simulink model "HW5_Q1_2sl"  (R2021b)
settings: Solver=VariableStepAuto  StartTime=0.0  StopTime=10.0  RelTol=1e-3
values from neighbouring files (symbols this model uses):
  Bm = 1*10^-5    (= 1e-05)    [HW5_Group3_1_1.m]    (also in HW5_Group3_1_2.m = 1e-08)
  Jm = 3*10^-5    (= 3e-05)    [HW5_Group3_1_1.m]    (also in HW5_Group3_1_2.m = 2.5e-05)
  Km = 3*10^-2    (= 0.03)    [HW5_Group3_1_1.m]    (also in HW5_Group3_1_2.m = 0.066)
  p = 3*10^-3    (= 0.003)    [HW5_Group3_1_2.m]    (also in HW5_Group3_3.m = 3)
  r = 10    [HW5_Group3_1_1.m]    (also in HW5_Group3_1_2.m = 6.25)
  Rm = 6    [HW5_Group3_1_1.m]    (also in HW5_Group3_1_2.m = 4.8)
  T_f = 0.023    [HW5_Group3_1_2.m]
libraries: SignalEditorBlockLib x1
settings Model: Creator=USER  LastModifiedBy=USER
settings DebuggingCC: UnconnectedInputMsg=none  UnconnectedOutputMsg=none  UnconnectedLineMsg=none
settings ModelReferenceCC: EnableRefExpFcnMdlSchedulingChecks=off
settings RTWCC: DLArmComputeVersion=20.02.1

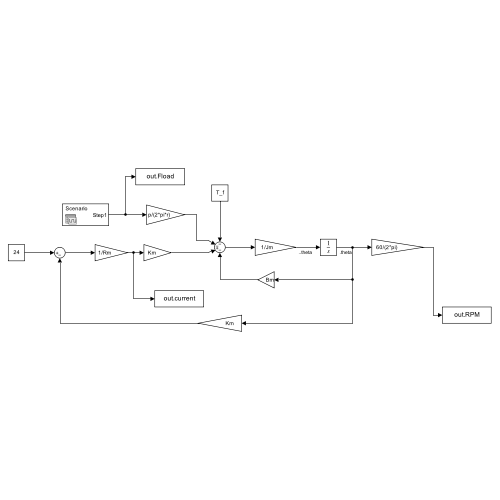
[thumbnail: Simulink's stored preview of the top-level diagram]
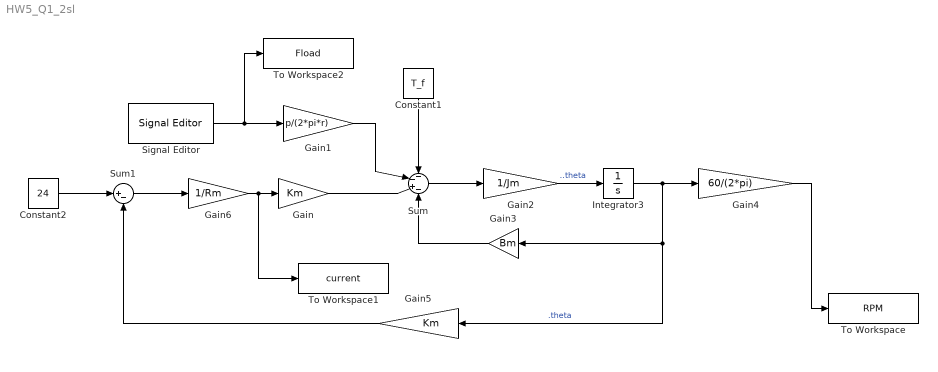
== system HW5_Q1_2sl ==
  Constant1 : Constant  Value=T_f
  Constant2 : Constant  Value=24
  Gain : Gain  Gain=Km
  Gain1 : Gain  Gain=p/(2*pi*r)
  Gain2 : Gain  Gain=1/Jm
  Gain3 : Gain  Gain=Bm
  Gain4 : Gain  Gain=60/(2*pi)
  Gain5 : Gain  Gain=Km
  Gain6 : Gain  Gain=1/Rm
  Integrator3 : Integrator
  Signal Editor : SignalEditorBlockLib/Signal Editor  FileName=C:\Users\USER\Desktop\大四上\SystemDynamic\112-1SystemDynammics\HW5_Group3\inputforce.mat  ActiveScenario=Scenario  ActiveSignal=Step1  IsBus=off  OutputBusObjectStr=Bus: BusObject  SampleTime=0  Interpolate=off  ZeroCross=off  OutputAfterFinalValue=Setting to zero  Unit=inherit  PreserveSignalName=on
  Sum : Sum  Inputs=--+-
  Sum1 : Sum  Inputs=|+-
  To Workspace : ToWorkspace  VariableName=RPM  SaveFormat=Timeseries  SampleTime=-1
  To Workspace1 : ToWorkspace  VariableName=current  SaveFormat=Timeseries  SampleTime=-1
  To Workspace2 : ToWorkspace  VariableName=Fload  SaveFormat=Timeseries  SampleTime=-1
  wires:
  Gain/1 -> Sum/3
  Gain1/1 -> Sum/2
  Signal Editor/1 -> To Workspace2/1, Gain1/1
  Sum/1 -> Gain2/1
  Gain2/1 -> Integrator3/1  "..theta"
  Integrator3/1 -> Gain4/1, Gain5/1, Gain3/1  ".theta"
  Gain3/1 -> Sum/4
  Gain4/1 -> To Workspace/1
  Constant1/1 -> Sum/1
  Gain5/1 -> Sum1/2
  Constant2/1 -> Sum1/1
  Sum1/1 -> Gain6/1
  Gain6/1 -> To Workspace1/1, Gain/1
